simulink model "SoC"  (R2025b)
settings: Solver=FixedStepAuto  StartTime=0.0  StopTime=100  FixedStep=0.01  RelTol=1e-3
libraries: simulink x1, SignalEditorBlockLib x1
settings Model: Creator=usuario  LastModifiedBy=usuario

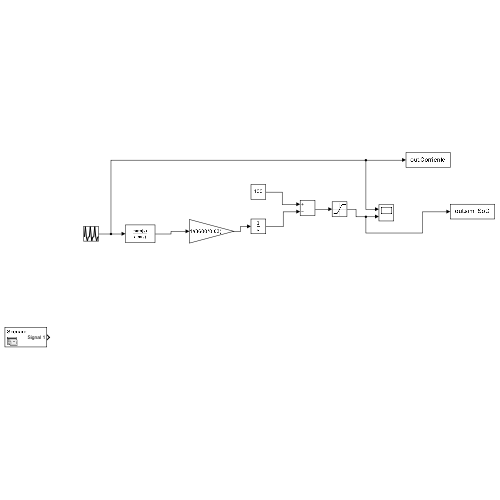
[thumbnail: Simulink's stored preview of the top-level diagram]
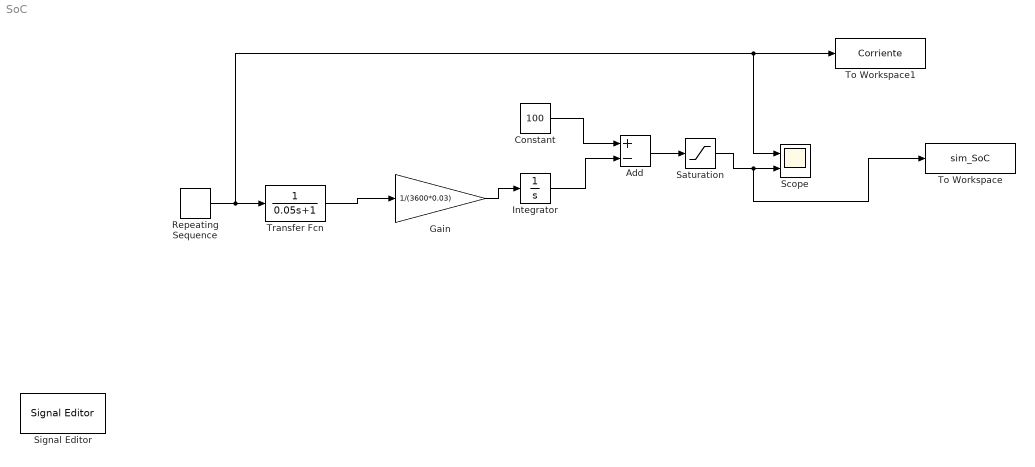
== system SoC ==
  Add : Sum  Inputs=+-
  Constant : Constant  Value=100
  Gain : Gain  Gain=1/(3600*0.03)
  Integrator : Integrator
  Repeating Sequence : simulink/Sources/Repeating Sequence  rep_seq_t=[0 2 4 6 8 10]  rep_seq_y=[0 100 0 -40 0 0]
  Saturation : Saturate  UpperLimit=100  LowerLimit=0
  Scope : Scope  NumInputPorts=2
      settings: ActiveDisplayYMinimum=-57.5  ActiveDisplayYMaximum=117.5
  Signal Editor : SignalEditorBlockLib/Signal Editor  FileName=Sis1.mat  ActiveScenario=Scenario  ActiveSignal=Signal 1  IsBus=off  OutputBusObjectStr=Bus: BusObject  SampleTime=0  ZeroCross=off  OutputAfterFinalValue=Setting to zero  Unit=inherit  PreserveSignalName=on  ApplySigPropsToAllScenarios=on  ApplySigPropsToAllSignals=off  SignalPropertySource=Dialog parameters
  To Workspace : ToWorkspace  VariableName=sim_SoC  SaveFormat=Timeseries  SampleTime=-1
  To Workspace1 : ToWorkspace  VariableName=Corriente  SaveFormat=Timeseries  SampleTime=-1
  Transfer Fcn : TransferFcn  Denominator=[0.05 1]
  wires:
  Gain/1 -> Integrator/1
  Constant/1 -> Add/1
  Integrator/1 -> Add/2
  Transfer Fcn/1 -> Gain/1
  Add/1 -> Saturation/1
  Saturation/1 -> To Workspace/1, Scope/2
  Repeating Sequence/1 -> Scope/1, To Workspace1/1, Transfer Fcn/1
